simulink model "PMSM_FOC_Average_Inveter"  (R2020b)
settings: Solver=FixedStepAuto  StartTime=0.0  StopTime=10  FixedStep=Fixed_Step_Size  RelTol=1e-3
model workspace (MAT data in the model file):
  wc = Simulink.Parameter
  wc.DataType = 'auto'
  wc.Dimensions = [0 0]
values from neighbouring files (symbols this model uses):
  Fixed_Step_Size = 2.5E-5    [Hall_Flux_FOC_Data.sldd]    (also in Motor_Control_Data.sldd = 1.0E-5
  Ld = 0.0004    [Hall_Flux_FOC_Data.sldd]    (also in Motor_Control_Data.sldd = 0.00014
  Lq = 0.00045    [Hall_Flux_FOC_Data.sldd]    (also in Motor_Control_Data.sldd = 0.0003115
  Pole_Pairs = 2.0    [Hall_Flux_FOC_Data.sldd]    (also in Motor_Control_Data.sldd = 4.0
undefined symbols (not defined in the file or in its folder): sigbuilder_block
libraries: simulink x1, mcbplantlib x1, autolibpmsminterior x1
settings Model: DataDictionary=Hall_Flux_FOC_Data.sldd  Creator=jt  LastModifiedBy=Administrator
settings DataIOCC: LimitDataPoints=on  SaveFormat=Array  ReturnWorkspaceOutputs=off
settings OptimizationCC: DefaultParameterBehavior=Inlined  UseDivisionForNetSlopeComputation=on  GainParamInheritBuiltInType=on  UseFloatMulNetSlope=on  InlineInvariantSignals=on  PassReuseOutputArgsAs=Individual arguments  ZeroExternalMemoryAtStartup=off  NoFixptDivByZeroProtection=on  EfficientFloat2IntCast=on  LifeSpan=1  OptimizeBlockOrder=speed  DifferentSizesBufferReuse=on  EfficientTunableParamExpr=on
settings DebuggingCC: AlgebraicLoopMsg=none  MaxConsecutiveZCsMsg=none  SolverPrmCheckMsg=warning  ParameterTunabilityLossMsg=error  AllowSymbolicDim=off  SFUnexpectedBacktrackingDiag=warning  SFNoUnconditionalDefaultTransitionDiag=warning  SFExecutionAtInitializationDiag=none  ArithmeticOperatorsInVariantConditions=warning
settings HardwareCC: ProdBitPerPointer=32  ProdBitPerSizeT=32  ProdBitPerPtrDiffT=32  ProdLargestAtomicInteger=Long  ProdLargestAtomicFloat=Double  ProdEndianess=BigEndian  ProdWordSize=32  ProdLongLongMode=on  ProdHWDeviceType=Freescale->32-bit PowerPC
settings ModelReferenceCC: PropagateSignalLabelsOutOfModel=off
settings SFSimCC: SimUseLocalCustomCode=off  SimParseCustomCode=off  MATLABDynamicMemAlloc=off  CustomCodeUndefinedFunction=UseInterfaceOnly
settings RTWCC: Description=Embedded Coder  SystemTargetFile=ert.tlc  GenCodeOnly=on  TemplateMakefile=ert_default_tmf  GenerateReport=on  RTWUseLocalCustomCode=off  IncludeHyperlinkInReport=on  LaunchReport=on  GenerateTraceInfo=on  GenerateTraceReport=on  GenerateTraceReportSl=on  GenerateTraceReportSf=on  GenerateTraceReportEml=on  GenerateCodeMetricsReport=on
settings CodeAppCC: ForceParamTrailComments=on  IgnoreCustomStorageClasses=off  OperatorAnnotations=on  SimulinkDataObjDesc=on  SFDataObjDesc=on  CustomSymbolStrGlobalVar=rt$N$M  CustomSymbolStrType=$N$M  CustomSymbolStrFcn=$N$M$F  CustomSymbolStrMacro=$N$M  InsertBlockDesc=on
settings ERTTargetCC: GenerateSampleERTMain=on  IncludeMdlTerminateFcn=off  CombineSignalStateStructs=on  SupportAbsoluteTime=off  SupportNonFinite=off  SupportComplex=off  SupportNonInlinedSFcns=on  InlinedParameterPlacement=NonHierarchical  ERTCustomFileTemplate=example_file_process.tlc
settings ConfigComp: CovMetricSettings=dw  CovSaveCumulativeToWorkspaceVar=on  CovSaveSingleToWorkspaceVar=on  CovExternalEMLEnable=off  CovSFcnEnable=off  PSAutoStubLUT=on  DVTestSuiteOptimization=Auto  DVDetectDeadLogic=on  DVDetectActiveLogic=on  DVDetectOutOfBounds=on  DVSaveReport=on  DVDisplayReport=off
settings SimscapeCC: SimscapeNormalizeSystem=off

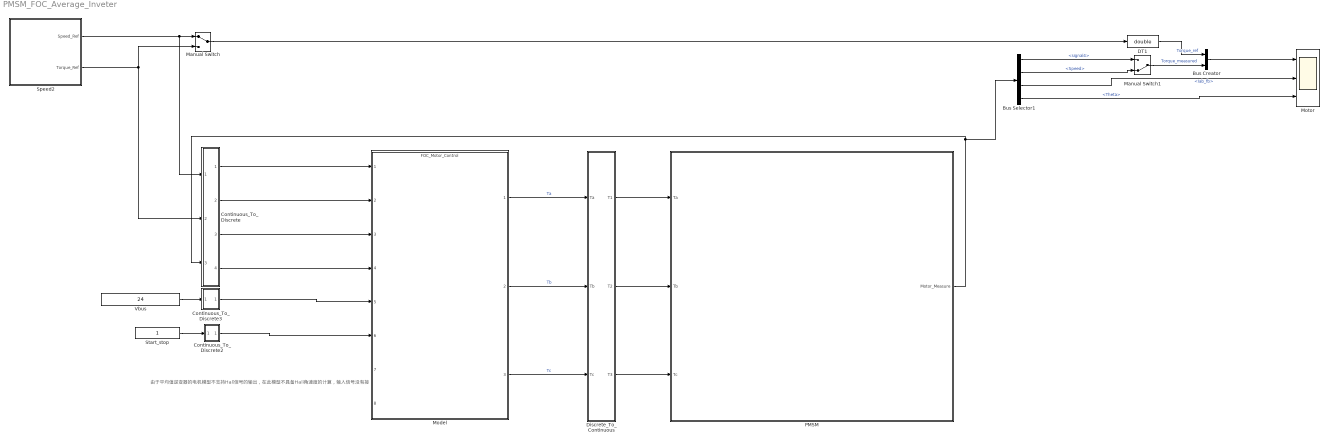
== system PMSM_FOC_Average_Inveter ==
  note: 由于平均值逆变器的电机模型不支持Hall信号的输出，在此模型不具备Hall角速度的计算，输入信号没有接
  Bus Creator : BusCreator  Inputs=2
  Bus Selector1 : BusSelector  OutputSignals=signal4,Speed,Iab_fb,Theta
  Continuous_To_Discrete : Subsystem
      mask Display: fprintf('C/D')
  Continuous_To_Discrete2 : Subsystem
      mask Display: fprintf('C/D')
  Continuous_To_Discrete3 : Subsystem
      mask Display: fprintf('C/D')
  DT1 : DataTypeConversion  OutDataTypeStr=double
  Discrete_To_Continuous : Subsystem  Description=""
      mask Display: fprintf('D/C')
  Manual Switch : ManualSwitch
  Manual Switch1 : ManualSwitch  CurrentSetting=0
  Model : ModelReference  ModelNameDialog=FOC_Motor_Control.slx  SimulationMode=Normal  CodeInterface=Top model  ModelReferenceVersion=1.61
  Motor : Scope  NumInputPorts=3
  PMSM : Subsystem
      mask Display: image('$imagefile'); % Use "Edit Image" on toolstrip to change.
  Speed2 : Subsystem  Tag=STV Subsys  LoadFcn=sigbuilder_block('load');  StartFcn=sigbuilder_block('start');  StopFcn=sigbuilder_block('stop');  ClipboardFcn=sigbuilder_block('clipboard');  mask(Sigbuilder block){tuvar=[0:10]}
      mask help: Simulink:masks:SigbuilderBlock_MD
      mask init:
      | if ~strcmp(get_param(bdroot(gcbh),'SimulationStatus'),'stopped') tuvar = sigbuilder_block('maskInit'); end
      settings: CopyFcn=sigbuilder_block('copy');  DeleteFcn=sigbuilder_block('delete');  ModelCloseFcn=sigbuilder_block('modelClose');  PreSaveFcn=sigbuilder_block('preSave');  PauseFcn=sigbuilder_block('pause');  ContinueFcn=sigbuilder_block('continue');  NameChangeFcn=sigbuilder_block('namechange');  OpenFcn=sigbuilder_block('open',[48.5 0 906 449 ]);  CloseFcn=sigbuilder_block('close');
      mask Display: plot(0, 0, 100, 100,[2, 2, 32, 32, 2], [68, 8, 8, 68, 68],[32, 2], [38, 38], [32, 19, 2],[53, 60, 44], [32, 17, 17, 2],[16, 16, 31, 31]);txt = getActiveGroup(gcbh);text(2, 100, txt,'verticalAlignment', 'top');
  Start_stop : Constant  OutDataTypeStr=uint8
  Vbus : Constant  Value=24  OutDataTypeStr=single
  wires:
  Discrete_To_Continuous/1(T1) -> PMSM/1(Ta)
  Discrete_To_Continuous/2(T2) -> PMSM/2(Tb)
  Discrete_To_Continuous/3(T3) -> PMSM/3(Tc)
  PMSM/1(Motor_Measure) -> Continuous_To_Discrete/3(Motor_Measurements), Bus Selector1/1
  Continuous_To_Discrete/4(Theta) -> Model/4
  Model/1 -> Discrete_To_Continuous/1(Ta)  "Ta"
  Model/2 -> Discrete_To_Continuous/2(Tb)  "Tb"
  Model/3 -> Discrete_To_Continuous/3(Tc)  "Tc"
  Bus Creator/1 -> Motor/1
  Bus Selector1/3 -> Motor/2  "<Iab_fb>"
  Speed2/1(Speed_Ref) -> Continuous_To_Discrete/1(Speed_Command), Manual Switch/1
  Continuous_To_Discrete/3(Phase_CurrentABC) -> Model/3
  Bus Selector1/4 -> Motor/3  "<Theta>"
  Start_stop/1 -> Continuous_To_Discrete2/1(Start_stop)
  Speed2/2(Torque_Ref) -> Continuous_To_Discrete/2(Torque_command), Manual Switch/2
  Manual Switch/1 -> DT1/1
  Bus Selector1/1 -> Manual Switch1/1  "<signal4>"
  Bus Selector1/2 -> Manual Switch1/2  "<Speed>"
  Manual Switch1/1 -> Bus Creator/2  "Torque_measured"
  Continuous_To_Discrete/2(Torque_ref) -> Model/2
  DT1/1 -> Bus Creator/1  "Torque_ref"
  Continuous_To_Discrete/1(Speed_target) -> Model/1
  Vbus/1 -> Continuous_To_Discrete3/1(Bus_Voltage)
  Continuous_To_Discrete3/1(Vbus) -> Model/5
  Continuous_To_Discrete2/1(Enable_Disable) -> Model/6

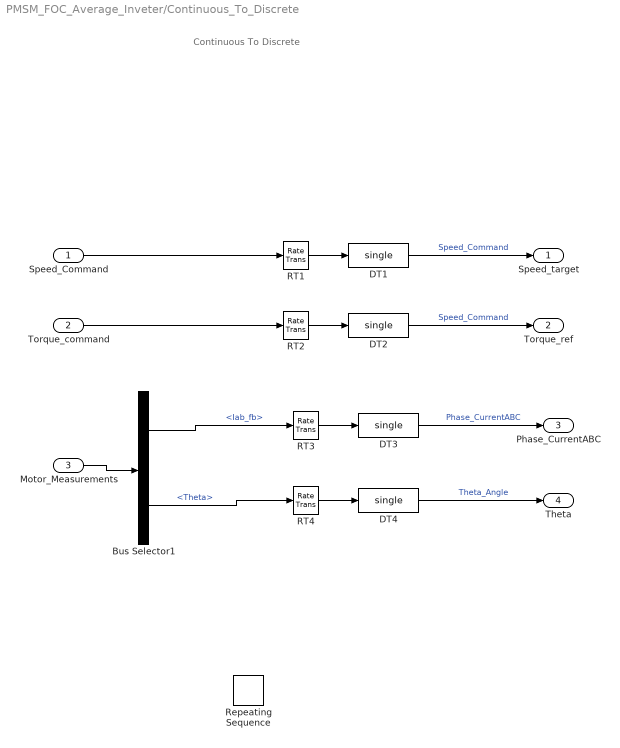
== system PMSM_FOC_Average_Inveter/Continuous_To_Discrete ==
  note: Continuous To Discrete
  Speed_Command : Inport
  Torque_command : Inport  Port=2
  Motor_Measurements : Inport  Port=3
  Bus Selector1 : BusSelector  OutputSignals=Iab_fb,Theta
  DT{1..4} (4 alike) : DataTypeConversion  OutDataTypeStr=single
  RT{1..4} (4 alike) : RateTransition  Integrity=off
  Repeating Sequence : simulink/Sources/Repeating Sequence  rep_seq_t=[0 0.1]  rep_seq_y=[0 6.28]
  Speed_target : Outport
  Torque_ref : Outport  Port=2
  Phase_CurrentABC : Outport  Port=3  PortDimensions=3
  Theta : Outport  Port=4
  wires:
  DT1/1 -> Speed_target/1  "Speed_Command"
  RT1/1 -> DT1/1
  RT3/1 -> DT3/1
  Motor_Measurements/1 -> Bus Selector1/1
  Speed_Command/1 -> RT1/1
  RT4/1 -> DT4/1
  DT4/1 -> Theta/1  "Theta_Angle"
  Bus Selector1/1 -> RT3/1  "<Iab_fb>"
  DT3/1 -> Phase_CurrentABC/1  "Phase_CurrentABC"
  Bus Selector1/2 -> RT4/1  "<Theta>"
  Torque_command/1 -> RT2/1
  RT2/1 -> DT2/1
  DT2/1 -> Torque_ref/1  "Speed_Command"

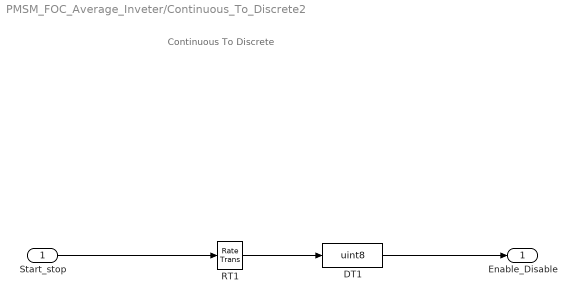
== system PMSM_FOC_Average_Inveter/Continuous_To_Discrete2 ==
  note: Continuous To Discrete
  Start_stop : Inport
  DT1 : DataTypeConversion  OutDataTypeStr=uint8
  RT1 : RateTransition  Integrity=off
  Enable_Disable : Outport
  wires:
  DT1/1 -> Enable_Disable/1
  RT1/1 -> DT1/1
  Start_stop/1 -> RT1/1

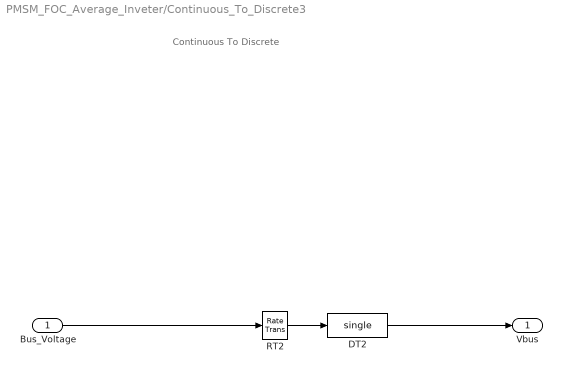
== system PMSM_FOC_Average_Inveter/Continuous_To_Discrete3 ==
  note: Continuous To Discrete
  Bus_Voltage : Inport
  DT2 : DataTypeConversion  OutDataTypeStr=single
  RT2 : RateTransition  Integrity=off
  Vbus : Outport
  wires:
  Bus_Voltage/1 -> RT2/1
  RT2/1 -> DT2/1
  DT2/1 -> Vbus/1

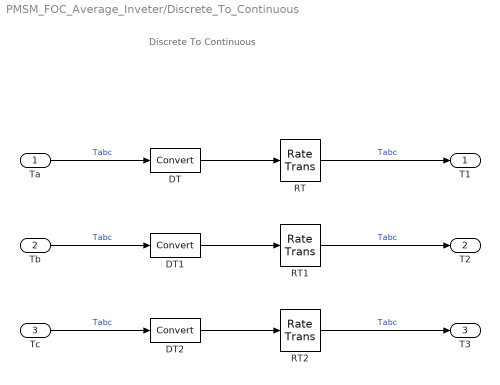
== system PMSM_FOC_Average_Inveter/Discrete_To_Continuous ==
  note: Discrete To Continuous
  Ta : Inport
  Tb : Inport  Port=2
  Tc : Inport  Port=3
  DT : DataTypeConversion
  DT1 : DataTypeConversion
  DT2 : DataTypeConversion
  RT : RateTransition  Integrity=off
  RT1 : RateTransition  Integrity=off
  RT2 : RateTransition  Integrity=off
  T1 : Outport
  T2 : Outport  Port=2
  T3 : Outport  Port=3
  wires:
  DT/1 -> RT/1
  Ta/1 -> DT/1  "Tabc"
  DT1/1 -> RT1/1
  Tb/1 -> DT1/1  "Tabc"
  DT2/1 -> RT2/1
  Tc/1 -> DT2/1  "Tabc"
  RT/1 -> T1/1  "Tabc"
  RT1/1 -> T2/1  "Tabc"
  RT2/1 -> T3/1  "Tabc"

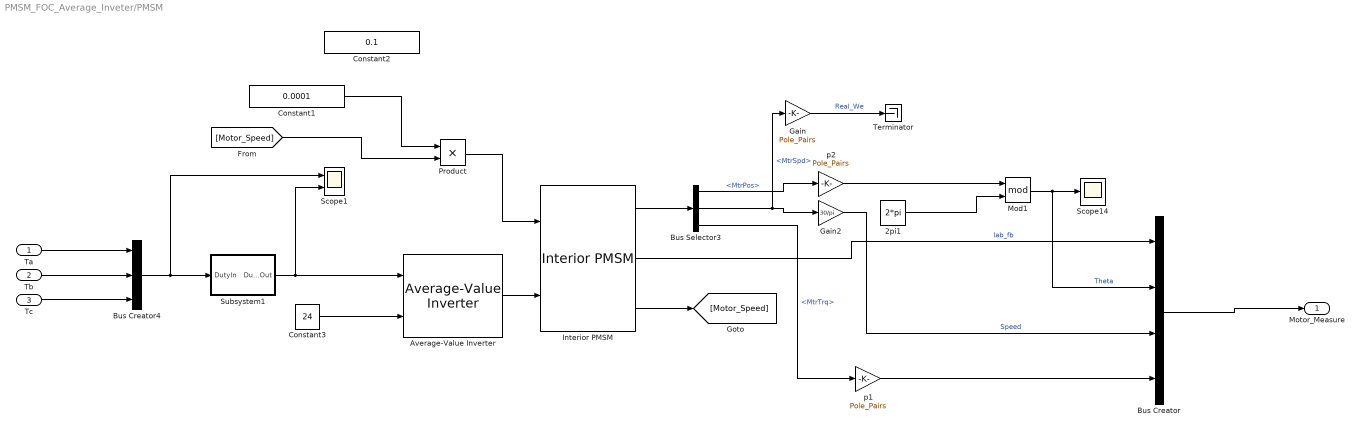
== system PMSM_FOC_Average_Inveter/PMSM ==
  Ta : Inport
  Tb : Inport  Port=2
  Tc : Inport  Port=3
  2pi1 : Constant  Value=2*pi
  Average-Value Inverter : mcbplantlib/Average-Value Inverter
  Bus Creator : BusCreator  Inputs=4
  Bus Creator4 : BusCreator  Inputs=3
  Bus Selector3 : BusSelector  OutputSignals=MtrPos,MtrSpd,MtrTrq
  Constant1 : Constant  Value=0.0001
  Constant2 : Constant  Value=0.1
  Constant3 : Constant  Value=24
  Gain : Gain  Gain=Pole_Pairs
  Gain2 : Gain  Gain=30/pi  OutDataTypeStr=Inherit: Same as input  ParamDataTypeStr=Inherit: Same as input
  Interior PMSM : autolibpmsminterior/Interior PMSM  port_config=Torque  sim_type=Discrete  Ts=Fixed_Step_Size  P=Pole_Pairs  Rs=R  Ldq=[Ld Lq]  KConstText=Permanent flux linkage constant (lambda_pm):  lambda_pm=Flux  Ke=159.9771  mechanical=[0.5e-4,8e-5,0]  idq0=[0 0]  theta_init=0  omega_init=0  KConst=Flux  lambda_pm_calc=Flux  Kt=0.07  RefBlkName='autolibpmsminterior/Interior PMSM'  aMode=5
      settings: SourceProductBaseCode=PW,MT,UV,VE,VP
  Mod1 : Math  Operator=mod  SaturateOnIntegerOverflow=on
  Product : Product
  Scope1 : Scope  NumInputPorts=2
  Scope14 : Scope
  Subsystem1 : Subsystem
  Terminator : Terminator
  p1 : Gain  Gain=Pole_Pairs  OutDataTypeStr=Inherit: Same as input  ParamDataTypeStr=Inherit: Same as input
  p2 : Gain  Gain=Pole_Pairs  OutDataTypeStr=Inherit: Same as input  ParamDataTypeStr=Inherit: Same as input
  Motor_Measure : Outport
  wires:
  Mod1/1 -> Bus Creator/2, Scope14/1  "Theta"
  Bus Creator/1 -> Motor_Measure/1
  Tc/1 -> Bus Creator4/3
  Interior PMSM/1 -> Bus Selector3/1
  Average-Value Inverter/1 -> Interior PMSM/2
  Subsystem1/1(DutyOut) -> Scope1/2, Average-Value Inverter/1
  Constant3/1 -> Average-Value Inverter/2
  Interior PMSM/2 -> Bus Creator/1  "Iab_fb"
  Bus Creator4/1 -> Subsystem1/1(DutyIn), Scope1/1
  Bus Selector3/2 -> Gain/1, Gain2/1  "<MtrSpd>"
  Bus Selector3/1 -> p2/1  "<MtrPos>"
  p2/1 -> Mod1/1
  2pi1/1 -> Mod1/2
  Gain2/1 -> Bus Creator/3  "Speed"
  Ta/1 -> Bus Creator4/1
  Tb/1 -> Bus Creator4/2
  Interior PMSM/3 -> [Motor_Speed]
  Bus Selector3/3 -> p1/1  "<MtrTrq>"
  p1/1 -> Bus Creator/4
  [Motor_Speed] -> Product/2
  Constant1/1 -> Product/1
  Product/1 -> Interior PMSM/1
  Gain/1 -> Terminator/1  "Real_We"

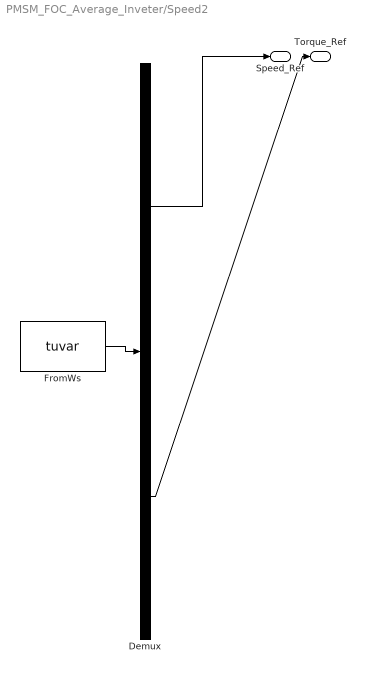
== system PMSM_FOC_Average_Inveter/Speed2 ==
  Demux : Demux  Tag=STV Demux  Outputs=2
      settings: DisplayOption=none
  FromWs : FromWorkspace  Tag=STV FromWs  VariableName=tuvar
      SigBuilderData=|
      | common.afterFinalStr = 'Extrapolate'
      | common.sampleTime = 0
      | dataSet.timeRange = [0 10]
      | dataSet.name = 'Target Speed'
      | sbobj.Groups.Name = 'Target Speed'
      | sbobj.Groups.Signals(1).Name = 'Speed_Ref'
      | sbobj.Groups.Signals(1).XData = [0 1 2.01 2.01 3 4.51 5.97 5.97 6.99 6.99 8.05 8.05 10]
      | sbobj.Groups.Signals(1).YData = [2005 2005 2005 2000 2000 2000 2000 1995 1995 2005 2005 2000 2000]
      | sbobj.Groups.Signals(2).Name = 'Torque_Ref'
      | sbobj.Groups.Signals(2).XData = [0 1.26 1.26 2.9 2.9 4.16 4.16 5.44 5.44 7.94 10]
      | sbobj.Groups.Signals(2).YData = [1 1 1.55 1.55 2.35 2.35 2.95 2.95 1.05 1.05 1.05]
  Speed_Ref : Outport  Tag=STV Outport
  Torque_Ref : Outport  Tag=STV Outport  Port=2
  wires:
  FromWs/1 -> Demux/1
  Demux/1 -> Speed_Ref/1
  Demux/2 -> Torque_Ref/1

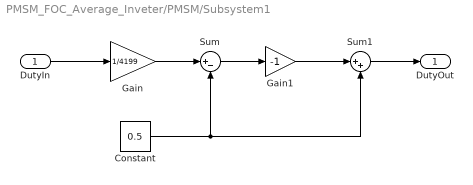
== system PMSM_FOC_Average_Inveter/PMSM/Subsystem1 ==
  DutyIn : Inport
  Constant : Constant  Value=0.5  SampleTime=-1
  Gain : Gain  Gain=1/4199  ParamDataTypeStr=single
  Gain1 : Gain  Gain=-1
  Sum : Sum  Inputs=|+-
  Sum1 : Sum  Inputs=|++
  DutyOut : Outport
  wires:
  Sum/1 -> Gain1/1
  Constant/1 -> Sum1/2, Sum/2
  DutyIn/1 -> Gain/1
  Gain1/1 -> Sum1/1
  Gain/1 -> Sum/1
  Sum1/1 -> DutyOut/1
